simulink library "lib_Gimbal_Cmd"  (R2018b)
settings: Solver=VariableStepAuto  StartTime=0.0  StopTime=10.0  RelTol=1e-3
settings Model: Creator=m.hiepp  LastModifiedBy=m.hiepp

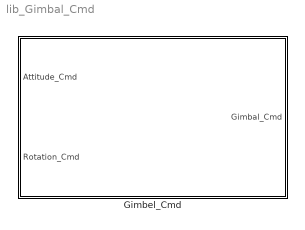
== system lib_Gimbal_Cmd ==
  Gimbel_Cmd : Subsystem

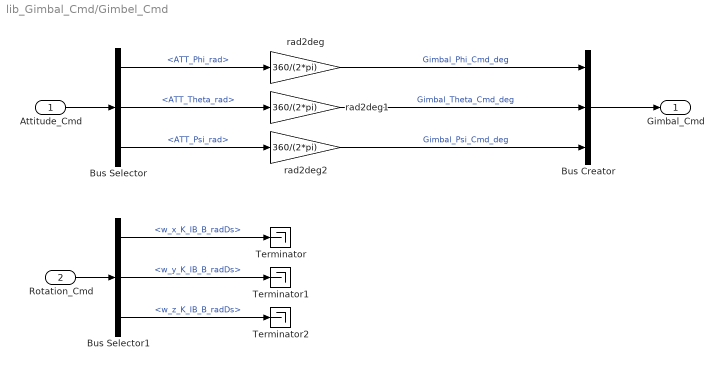
== system lib_Gimbal_Cmd/Gimbel_Cmd ==
  Attitude_Cmd : Inport  OutDataTypeStr=Bus: Attitude_States_Bus
  Rotation_Cmd : Inport  Port=2  OutDataTypeStr=Bus: Rotation_States_Bus
  Bus Creator : BusCreator  Inputs=3  OutDataTypeStr=Bus: Gimbal_Cmd_Bus
  Bus Selector : BusSelector  OutputSignals=ATT_Euler.ATT_Phi_rad,ATT_Euler.ATT_Theta_rad,ATT_Euler.ATT_Psi_rad
  Bus Selector1 : BusSelector  OutputSignals=w_x_K_IB_B_radDs,w_y_K_IB_B_radDs,w_z_K_IB_B_radDs
  Terminator : Terminator
  Terminator1 : Terminator
  Terminator2 : Terminator
  rad2deg : Gain  Gain=360/(2*pi)
  rad2deg1 : Gain  Gain=360/(2*pi)
  rad2deg2 : Gain  Gain=360/(2*pi)
  Gimbal_Cmd : Outport  OutDataTypeStr=Bus: Gimbal_Cmd_Bus
  wires:
  Attitude_Cmd/1 -> Bus Selector/1
  Bus Selector/1 -> rad2deg/1  "<ATT_Phi_rad>"
  Bus Selector/2 -> rad2deg1/1  "<ATT_Theta_rad>"
  Bus Selector/3 -> rad2deg2/1  "<ATT_Psi_rad>"
  rad2deg/1 -> Bus Creator/1  "Gimbal_Phi_Cmd_deg"
  rad2deg1/1 -> Bus Creator/2  "Gimbal_Theta_Cmd_deg"
  rad2deg2/1 -> Bus Creator/3  "Gimbal_Psi_Cmd_deg"
  Bus Creator/1 -> Gimbal_Cmd/1
  Rotation_Cmd/1 -> Bus Selector1/1
  Bus Selector1/1 -> Terminator/1  "<w_x_K_IB_B_radDs>"
  Bus Selector1/2 -> Terminator1/1  "<w_y_K_IB_B_radDs>"
  Bus Selector1/3 -> Terminator2/1  "<w_z_K_IB_B_radDs>"
